simulink model "PV_Inverter"  (R2023a)
settings: Solver=VariableStepAuto  StartTime=0.0  StopTime=2  RelTol=1e-3
libraries: spsMosfetLib x5, spsRMSLib x5, spsSeriesRLCBranchLib x4, spsVoltageMeasurementLib x3, spsDiodeLib x2, spsPWMGeneratorDCDCLib x2, spsCurrentMeasurementLib x2, spsLinearTransformerLib x1, slpidlib x1, spsPVArrayLib x1, spspowerguiLib x1
settings Model: Creator=mnith  LastModifiedBy=mnith

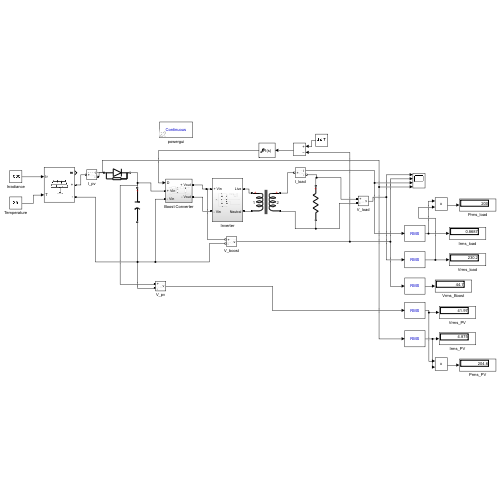
[thumbnail: Simulink's stored preview of the top-level diagram]
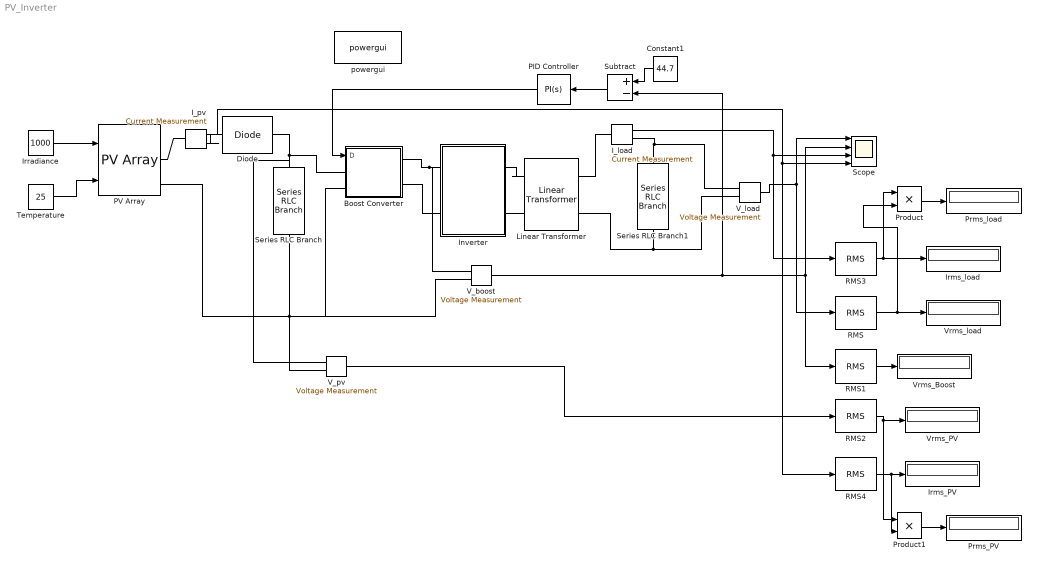
== system PV_Inverter ==
  Boost Converter : Subsystem
  Constant1 : Constant  Value=44.7
  Diode : spsDiodeLib/Diode  Ron=0.001  Lon=0  Vf=0  IC=0  UseSnubber=0  Rs=500  Cs=250e-9  Measurements=off
  I_load : spsCurrentMeasurementLib/Current Measurement  PhasorSimulation=off  OutputType=Complex  PSBequivalent=0
  I_pv : spsCurrentMeasurementLib/Current Measurement  PhasorSimulation=off  OutputType=Complex  PSBequivalent=0
  Inverter : Subsystem
  Irms_PV : Display
  Irms_load : Display
  Irradiance : Constant  Value=1000
  Linear Transformer : spsLinearTransformerLib/Linear Transformer  UNITS=SI  NominalPower=[ 300 50 ]  winding1=[44.7 0 0]  winding2=[235 0 0]  ThreeWindings=off  winding3=[3.15e+05 6.615e+05 84225]  RmLm=[inf inf]  Measurements=None  DataType=on
  PID Controller : slpidlib/PID Controller  Controller=PI  Form=Parallel  TimeDomain=Continuous-time  UseExternalTs=off  SampleTime=-1  IntegratorMethod=Forward Euler  FilterMethod=Forward Euler  ControllerParametersSource=internal  P=0.023  I=1  UseKiTs=off  D=0  N=100  UseFilter=on  TunerSelectOption=Transfer Function Based (PID Tuner App)  InitialConditionSource=internal  InitialConditionForIntegrator=0  InitialConditionForFilter=0  DifferentiatorICPrevScaledInput=0  ExternalReset=none  TrackingMode=off  Kt=1  LimitOutput=on  SatLimitsSource=internal  UpperSaturationLimit=0.16  LowerSaturationLimit=0  LinearizeAsGain=on  AntiWindupMode=none  Kb=1  LimitIntegrator=on  UpperIntegratorSaturationLimit=0.16  LowerIntegratorSaturationLimit=-0.16  POutMin=[]  POutMax=[]  IOutMin=[]  IOutMax=[]  DOutMin=[]  DOutMax=[]  NOutMin=[]  NOutMax=[]  SumOutMin=[]  SumOutMax=[]  SaturationOutMin=[]  SaturationOutMax=[]  PParamMin=[]  PParamMax=[]  IParamMin=[]  IParamMax=[]  DParamMin=[]  DParamMax=[]  NParamMin=[]  NParamMax=[]  KbParamMin=[]  KbParamMax=[]  KtParamMin=[]  KtParamMax=[]  KbOutMin=[]  KbOutMax=[]  KtOutMin=[]  KtOutMax=[]  IntegratorOutMin=[]  IntegratorOutMax=[]  FilterOutMin=[]  FilterOutMax=[]  SumI1OutMin=[]  SumI1OutMax=[]  SumI2OutMin=[]  SumI2OutMax=[]  SumI3OutMin=[]  SumI3OutMax=[]  SumI4OutMin=[]  SumI4OutMax=[]  SumDOutMin=[]  SumDOutMax=[]  DifferentiatorOutMin=[]  DifferentiatorOutMax=[]  FilterDiffOutCoefMin=[]  FilterDiffOutCoefMax=[]  ReciprocalOutMin=[]  ReciprocalOutMax=[]  SumDenOutMin=[]  SumDenOutMax=[]  SumNumOutMin=[]  SumNumOutMax=[]  DivideOutMin=[]  DivideOutMax=[]  UdiffTsProdOutMin=[]  UdiffTsProdOutMax=[]  NTsProdOutMin=[]  NTsProdOutMax=[]  UintegralTsProdOutMin=[]  UintegralTsProdOutMax=[]  UngainTsProdOutMin=[]  UngainTsProdOutMax=[]  ClampingZeroOutDataTypeStr=Inherit: Inherit via back propagation  ClampingZeroOutMin=[]  ClampingZeroOutMax=[]  FilterDenConstantOutDataTypeStr=Inherit: Inherit via back propagation  FilterDenConstantOutMin=[]  FilterDenConstantOutMax=[]  PCopyOutDataTypeStr=Inherit: Inherit via back propagation  PCopyOutMin=[]  PCopyOutMax=[]  NCopyOutDataTypeStr=Inherit: Inherit via back propagation  NCopyOutMin=[]  NCopyOutMax=[]  IntegratorContinuousStateAttributes=''  IntegratorStateMustResolveToSignalObject=off  IntegratorRTWStateStorageClass=Auto  FilterContinuousStateAttributes=''  FilterStateMustResolveToSignalObject=off  FilterRTWStateStorageClass=Auto  ParallelPVariant=InternalParameters  IdealPVariant=Disabled  IVariant=InternalParameters  DVariant=Disabled  IntegratorVariant=Continuous  SatVariant=Enabled  AWVariant=Passthrough  PCopyVariant=Disabled  TRVariant=Disabled  FdbkBlocksVariant=Forward  IdealPFdbkVariant=Disabled  SatFdbkVariant=Disabled  DerivativeFilterVariant=Disabled  NVariant=Disabled  NCopyVariant=Disabled_SignalSpec  FilterICVariant=Disabled  IntegratorICVariant=InternalICs  ExternalResetVariant=Disabled  TRSumVariant=Passthrough  SumFdbkVariant=Disabled  SumVariant=Sum_PI  TsampFilterVariant=InternalTs  TsampNgainVariant=Passthrough  TsampIntegralVariant=Disabled_SignalSpec  ExternalSaturationOutDataTypeStr=Inherit: Same as second input
  PV Array : spsPVArrayLib/PV Array  Npar=1  Nser=1  PlotType=one module @ 25 deg.C & specified irradiances  S_vec="[ 1000  800 600 400 200 ]"  Temp_C_vec=[ 10 25 40 55 70 ]  ModuleName=User-defined  PlotWhenSelected=off  Pm=300.0738  Ncell=72  Voc=44.71  Isc=8.947  Vm=37.23  Im=8.06  beta_Voc_pc=-0.34  alpha_Isc_pc=0.102  beta_Voc=-0.15201  alpha_Isc=0.0091259  IL=8.9758  I0=1.5571e-10  nI=0.97821  Rsh=74.2964  Rs=0.23882  RobustModel=off  RobustCellTemperature=313.3991  BAL=on  Tc=1e-6  Tfilter=5e-5
  Prms_PV : Display
  Prms_load : Display
  Product : Product
  Product1 : Product
  RMS{,1..4} (5 alike) : spsRMSLib/RMS  TrueRMS=on  Freq=60  RMSInit=120  Ts=0
  Scope : Scope  NumInputPorts=4
  Series RLC Branch : spsSeriesRLCBranchLib/Series RLC Branch  LConnTagsString=__new0  RConnTagsString=__new0  BranchType=C  Resistance=1  Inductance=1e-3  SetiL0=off  InitialCurrent=0  Capacitance=1e-3  Setx0=off  InitialVoltage=0  Measurements=None
  Series RLC Branch1 : spsSeriesRLCBranchLib/Series RLC Branch  LConnTagsString=__new0  RConnTagsString=__new0  BranchType=R  Resistance=265  Inductance=1e-3  SetiL0=off  InitialCurrent=0  Capacitance=1e-6  Setx0=off  InitialVoltage=0  Measurements=None
  Subtract : Sum  Inputs=+-
  Temperature : Constant  Value=25
  V_boost : spsVoltageMeasurementLib/Voltage Measurement  PhasorSimulation=off  OutputType=Complex  PSBequivalent=0
  V_load : spsVoltageMeasurementLib/Voltage Measurement  PhasorSimulation=off  OutputType=Complex  PSBequivalent=0
  V_pv : spsVoltageMeasurementLib/Voltage Measurement  PhasorSimulation=off  OutputType=Complex  PSBequivalent=0
  Vrms_Boost : Display
  Vrms_PV : Display
  Vrms_load : Display
  powergui : spspowerguiLib/powergui  Priority=1  SimulationMode=Continuous  SampleTime=5e-6  frequency=60  Iterations=50  frequencyindice=0  Pbase=100e6  ErrMax=1e-4  UnitsV=kV  UnitsW=MW  buscounter=0  FunctionMessages=off  echomessages=off  EnableUseOfTLC=off  CurrentSourceSwitches=off  DisableSnubberDevices=off  DisableRonSwitches=off  DisableVfSwitches=off  DisplayEquations=off  AutomaticDiscreteSolvers=off  SolverType=Tustin/Backward Euler (TBE)  Interpol=off  ExternalGateDelay=off  methode=off  Ts=100  x0status=blocks  SPID=on  SwTol=0  HookPort=off  NonlinearTolerance=1e-4  nMaxIteration=100  ContinueOnMaxIteration=off  RestoreLinks=warning  ResistiveCurrentMeasurement=off  Frange=[0:2:500]  Ylog=off  Xlog=on  ShowGrid=off  save=off  variable=ZData  structure=0  ZoomFFT=off  StartTime=0.0  cycles=1  DisplayStyle=1  fundamental=60  FreqAxis=off  MaxFrequency=1000  frequencyindicesteady=1  RmsSteady=1  display=off
  wires:
  Irradiance/1 -> PV Array/1
  Temperature/1 -> PV Array/2
  V_load/1 -> RMS/1, Scope/1
  V_boost/1 -> Subtract/2, RMS1/1, Scope/2
  I_load/1 -> RMS3/1, Scope/3
  I_pv/1 -> RMS4/1, Scope/4
  RMS/1 -> Product/2, Vrms_load/1
  RMS1/1 -> Vrms_Boost/1
  RMS3/1 -> Product/1, Irms_load/1
  Product/1 -> Prms_load/1
  Product1/1 -> Prms_PV/1
  RMS2/1 -> Vrms_PV/1, Product1/1
  RMS4/1 -> Irms_PV/1, Product1/2
  V_pv/1 -> RMS2/1
  Subtract/1 -> PID Controller/1
  Constant1/1 -> Subtract/1
  PID Controller/1 -> Boost Converter/1(D)
  connections:
  PV Array/RConn2 -- V_boost/LConn2 -- Boost Converter/LConn2 -- V_pv/LConn2 -- Series RLC Branch/RConn1
  Linear Transformer/LConn1 -- Inverter/RConn1
  V_load/LConn1 -- I_load/RConn1 -- Series RLC Branch1/LConn1
  Linear Transformer/RConn2 -- V_load/LConn2 -- Series RLC Branch1/RConn1
  I_load/LConn1 -- Linear Transformer/RConn1
  I_pv/RConn1 -- Diode/LConn1
  I_pv/LConn1 -- PV Array/RConn1
  Inverter/RConn2 -- Linear Transformer/LConn2
  Diode/RConn1 -- Boost Converter/LConn1 -- V_pv/LConn1 -- Series RLC Branch/LConn1
  Inverter/LConn2 -- Boost Converter/RConn2
  Inverter/LConn1 -- Boost Converter/RConn1 -- V_boost/LConn1

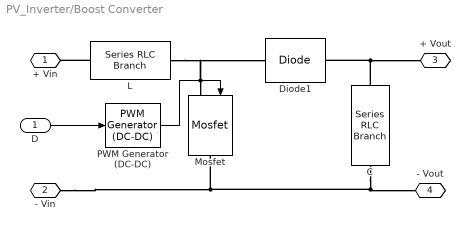
== system PV_Inverter/Boost Converter ==
  D : Inport
  C : spsSeriesRLCBranchLib/Series RLC Branch  LConnTagsString=__new0  RConnTagsString=__new0  BranchType=C  Resistance=1  Inductance=1e-3  SetiL0=off  InitialCurrent=0  Capacitance=2.66e-3  Setx0=off  InitialVoltage=0  Measurements=None
  Diode1 : spsDiodeLib/Diode  Ron=0.001  Lon=0  Vf=0  IC=0  UseSnubber=0  Rs=500  Cs=250e-9  Measurements=off
  L : spsSeriesRLCBranchLib/Series RLC Branch  LConnTagsString=__new0  RConnTagsString=__new0  BranchType=L  Resistance=10  Inductance=12.36e-3  SetiL0=off  InitialCurrent=0  Capacitance=1e-6  Setx0=off  InitialVoltage=0  Measurements=None
  Mosfet : spsMosfetLib/Mosfet  Ron=0.1  Lon=0  Rd=0.01  Vfd=0  IC=0  Rs=1e5  Cs=inf  Measurements=off
  PWM Generator (DC-DC) : spsPWMGeneratorDCDCLib/PWM Generator (DC-DC)  Fsw=5000  Ts=0
  + Vin : PMIOPort  Side=Left
  - Vin : PMIOPort  Port=2  Side=Left
  + Vout : PMIOPort  Port=3  Side=Right
  - Vout : PMIOPort  Port=4  Side=Right
  wires:
  D/1 -> PWM Generator (DC-DC)/1
  PWM Generator (DC-DC)/1 -> Mosfet/1
  connections:
  C/LConn1 -- Diode1/RConn1 -- + Vout/RConn1
  Mosfet/LConn1 -- L/RConn1 -- Diode1/LConn1
  C/RConn1 -- - Vout/RConn1 -- Mosfet/RConn1 -- - Vin/RConn1
  L/LConn1 -- + Vin/RConn1

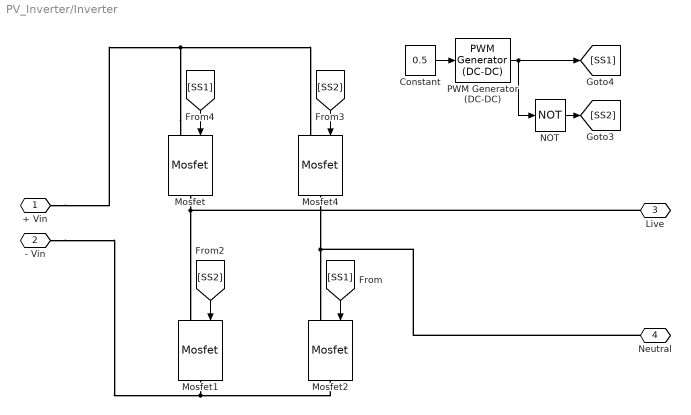
== system PV_Inverter/Inverter ==
  Constant : Constant  Value=0.5
  Mosfet{,1..2,4} (4 alike) : spsMosfetLib/Mosfet  Ron=0.1  Lon=0  Rd=0.01  Vfd=0  IC=0  Rs=1e5  Cs=inf  Measurements=off
  NOT : Logic  Operator=NOT  IconShape=distinctive  AllPortsSameDT=off  OutDataTypeStr=boolean
  PWM Generator (DC-DC) : spsPWMGeneratorDCDCLib/PWM Generator (DC-DC)  Fsw=50  Ts=0
  + Vin : PMIOPort  Side=Left
  - Vin : PMIOPort  Port=2  Side=Left
  Live : PMIOPort  Port=3  Side=Right
  Neutral : PMIOPort  Port=4  Side=Right
  wires:
  [SS1] -> Mosfet/1
  [SS2] -> Mosfet4/1
  [SS1] -> Mosfet2/1
  [SS2] -> Mosfet1/1
  PWM Generator (DC-DC)/1 -> [SS1], NOT/1
  NOT/1 -> [SS2]
  Constant/1 -> PWM Generator (DC-DC)/1
  connections:
  Mosfet1/RConn1 -- - Vin/RConn1 -- Mosfet2/RConn1
  Mosfet/RConn1 -- Live/RConn1 -- Mosfet1/LConn1
  Mosfet/LConn1 -- + Vin/RConn1 -- Mosfet4/LConn1
  Mosfet4/RConn1 -- Neutral/RConn1 -- Mosfet2/LConn1
